simulink model "ultra"  (R2020b)
settings: Solver=FixedStepDiscrete  StartTime=0.0  StopTime=10.0  FixedStep=0.0005  RelTol=1e-3  EnableMultiTasking=on
undefined symbols (not defined in the file): acc_calmax1, acc_calmax2, acc_calmin1, acc_calmin2, akemancanshu, bre, bre_calmax, bre_calmin, ecucoder_acal, I_AN01_5K1, I_AN03_5V, I_AN04_5V, kd, ki, kp, leftmax, O_SW06_HS1A, rightmax, T_add, T_del, tiaoshi, zhiling
libraries: ec5744lib x215, canmsglib x75, simulink x10
(part 7 of 7)

== matlab function ultra/run/ctrl/Subsystem1/control_strategy/MATLAB Function ==
  data: slip_ratio_fl input; torque_cmd_fl output; slip_ratio_fr input; slip_ratio_rl input; slip_ratio_rr input; desired_slip_ratio input; driver_torque_cmd_fl input; driver_torque_cmd_fr input; driver_torque_cmd_rl input; driver_torque_cmd_rr input; dt input; B input; C input; D input; E input; wheel_radius input; torque_cmd_fr output; torque_cmd_rl output; torque_cmd_rr output
function [torque_cmd_fl, torque_cmd_fr, torque_cmd_rl, torque_cmd_rr] = SlipRatioControlWithMagicFormula(slip_ratio_fl, slip_ratio_fr, slip_ratio_rl, slip_ratio_rr, desired_slip_ratio, driver_torque_cmd_fl, driver_torque_cmd_fr, driver_torque_cmd_rl, driver_torque_cmd_rr, dt, B, C, D, E, wheel_radius)

    % 定义持久变量来存储每个轮胎的上一次误差
    persistent e_prev_fl e_prev_fr e_prev_rl e_prev_rr
    if isempty(e_prev_fl)
        e_prev_fl = 0; e_prev_fr = 0; e_prev_rl = 0; e_prev_rr = 0;
    end

    % 滑膜设计参数
    lambda = 2;            
    K = 0.2;               
    delta = 0.05;          

    % 定义一个内部函数来为每个轮胎进行滑膜控制
    function [torque_cmd, e_prev] = singleWheelControl(slip_ratio, desired_slip_ratio, driver_torque_cmd, e_prev, B, C, D, E, wheel_radius)
        % 计算误差和误差的变化率
        e = desired_slip_ratio - slip_ratio;
        e_dot = (e - e_prev) / dt;
        s = e_dot + lambda * e;

        % 使用Magic Formula计算期望的轮胎纵向力
        Fx_desired = D * sin(C * atan(B * desired_slip_ratio - E*(B * desired_slip_ratio - atan(B * desired_slip_ratio))));
        
        % 转换纵向力为期望扭矩
        desired_torque = Fx_desired * wheel_radius;

        % 根据滑模控制策略调整扭矩
        if abs(s) < delta
            torque_adjustment = 0;
        else
            torque_adjustment = K * s;
        end

        % 结合Magic Formula期望扭矩和滑模控制调整来计算输出扭矩
        torque_cmd = desired_torque + torque_adjustment;
        
        % 保证输出扭矩为非负
        torque_cmd = max(0, torque_cmd); 

        % 更新误差以供下次使用
        e_prev = e;
    end

    % 为每个轮胎应用滑模控制策略
    [torque_cmd_fl, e_prev_fl] = singleWheelControl(slip_ratio_fl, desired_slip_ratio, driver_torque_cmd_fl, e_prev_fl, B, C, D, E, wheel_radius);
    [torque_cmd_fr, e_prev_fr] = singleWheelControl(slip_ratio_fr, desired_slip_ratio, driver_torque_cmd_fr, e_prev_fr, B, C, D, E, wheel_radius);
    [torque_cmd_rl, e_prev_rl] = singleWheelControl(slip_ratio_rl, desired_slip_ratio, driver_torque_cmd_rl, e_prev_rl, B, C, D, E, wheel_radius);
    [torque_cmd_rr, e_prev_rr] = singleWheelControl(slip_ratio_rr, desired_slip_ratio, driver_torque_cmd_rr, e_prev_rr, B, C, D, E, wheel_radius);

end

== matlab function ultra/无人TX/转向换算/MATLAB Function1 ==
  data: y1 output; y2 output; biaozhi2 output; baocuo input
function [y1,y2,biaozhi2] = fcn(baocuo)
    persistent i;
     % 初始化状态变量
    if isempty(i)
        i = 1;
    end
    if baocuo==1
        i=1;
    end
    if i<4
        biaozhi2=1;
    else
        biaozhi2=0;
    end
    if mod(i, 2) == 0
        result = 1;
    else
        result = 0;
    end
    
    if result==0
        y1=6307883;
        y2=0;
    else
        y1=6307883;
        y2=128;
    end
    i=i+1;

== matlab function ultra/TX控制器/速度/185右前/MATLAB Function1 ==
  data: v input; T output; a input
function T = fcn(v,a)
% if a>5
%     y = u;
% elseif a>3&&a<5
%     y=1200;
% else
%     y=800;
% end

if v<6000*1.88e-3
    T=2100;
elseif v>11000*1.88e-3
    T=800;
else
    T=1100;
end

== matlab function ultra/RX/287 289右后/Subsystem3/Subsystem/MATLAB Function ==
  data: u input; y output
function y = fcn(u)


y = u/594.06;

== matlab function ultra/TOWORKSTATION/转向/Subsystem/MATLAB Function1 ==
  data: y1 output; y2 output; biaozhi2 output
function [y1,y2,biaozhi2] = fcn()
    persistent i;
     % 初始化状态变量
    if isempty(i)
        i = 1;
    end
    if i<16
        biaozhi2=1;
    else
        biaozhi2=0;
    end
    if mod(i, 2) == 0
        result = 1;
    else
        result = 0;
    end
    
    if result==0
        y1=6307883;
        y2=0;
    else
        y1=6307883;
        y2=128;
    end
    i=i+1;

== matlab function ultra/TX控制器/速度/184左前/MATLAB Function ==
  data: u input; y output; zhidongesc input; zhidongebs input
function y = fcn(u,zhidongesc,zhidongebs)
 y = u*594.06;
if zhidongesc>1800&&zhidongebs==2
    y = u*594.06;
end
if zhidongesc<1500&&zhidongebs==2
    y=0;
end

== matlab function ultra/TX控制器/速度/185右前/MATLAB Function ==
  data: u input; y output; zhidongesc input; zhidongebs input
function y = fcn(u,zhidongesc,zhidongebs)
 y = u*594.06;
if zhidongesc>1800&&zhidongebs==2
    y = u*594.06;
end
if zhidongesc<1500&&zhidongebs==2
    y=0;
end

== matlab function ultra/TX控制器/速度/189左后/MATLAB Function ==
  data: u input; y output; zhidongesc input; zhidongebs input
function y = fcn(u,zhidongesc,zhidongebs)
 y = u*594.06;
if zhidongesc>1800&&zhidongebs==2
    y = u*594.06;
end
if zhidongesc<1500&&zhidongebs==2
    y=0;
end

== matlab function ultra/TX控制器/速度/185右前/MATLAB Function3 ==
  data: v input; y output; angle input; vz input; model input
function y = fcn(v, angle, vz,model)
if (angle>3||angle<-3)&&model==3%4650000,4870000,4741002
    y=vz*594.06;
else
    y = v;
end

== matlab function ultra/run/滑移率计算 ==
  data: vyouhou input; slipyuohou output; vyouqian input; vzouhou input; vzuoqian input; v input; slipyouqian output; slipzuohou output; slipzuoqian output; vmin input
function [slipyuohou,slipyouqian,slipzuohou,slipzuoqian] = fcn(vyouhou,vyouqian,vzouhou,vzuoqian,v,vmin)

    v1=vmin;
if v<0.1
    v1 = vmin;
else
    v1 = v;
end
slipyuohou= (vyouhou - v1) / vyouhou;
slipzuohou= (vzouhou - v1) / vzouhou;
slipyouqian= (vyouqian - v1) / vyouqian;
slipzuoqian= (vzuoqian - v1) / vzuoqian;
end

== matlab function ultra/TOWORKSTATION/转向/Subsystem/Subsystem/MATLAB Function ==
  data: steer output; y output
function [steer,y] = fcn()
  persistent i;
     % 初始化状态变量
    if isempty(i)
        i = 0;
    end
    x=0;
    if i>1
       steer=62000* sin(2 * pi * i)+683198;
%            steer= 3494 *x+2.407e+04 ;
%            x=(i-1)*50;
%            if i>8.2
%                i=1;
%            end
    else
        steer=683198
    end
%     if i>0.2     
%         steer=  3271 *x+6.821e+05 ;
% %         if x==0
% %             steer=25092;
% %         end
%     else
%         steer=683198;
%     end
    i=i+0.02;
  persistent time;
     % 初始化状态变量
    if isempty(time)
        time = 0;
    end
    if mod(time, 2) == 0
        result = 1;
    else
        result = 0;
    end
    if time<5
    y=6;
 
    elseif time>=5&&time<10
    y=15;
  
    elseif time>=10
        if result==1
            y=79;
        else
            y=63;
        end
    else
        y=6;
    end   
    time=time+1;
    if time>650
        y=6;
    end
end

== matlab function ultra/TX控制器/MATLAB Function1 ==
  data: y output; model input
function y = fcn(model)
if (model==1||model==2||model==3||model==4||model==5||model==6||model==7||model==8)
    y=1;
else
    y=0;
end

== matlab function ultra/run/ctrl/Subsystem1/control_strategy/差速/差速/pid ==
  data: v input; u input; v_zuoqian output
function v_zuoqian  = carPIDControl(v, u)
    % 赛车PID控制器参数
    kp = 0.2;
    ki = 0.1;
    kd = 0.01;
    
    % 状态变量
    persistent integral previous_error 
    
    % 初始化状态变量
    if isempty(integral)
        integral = 0;
        previous_error = 0;
        i=0;
    end
    
    % PID控制器计算
    error = u - v;
    integral = integral + error*0.02;
    derivative = (error - previous_error)/0.02;
    
        if integral > 0.4    
        integral = 0.4;
        end
        if integral < -0.4    
        integral = -0.4;
        end
    
   v_zuoqian = kp * error + ki * integral + kd * derivative;
   
    % 保存上一个误差用于下次计算
    previous_error = error;
end

== matlab function ultra/run/ctrl/Subsystem1/control_strategy/差速/差速/pid1 ==
  data: v input; u input; v_zuoqian output
function v_zuoqian  = carPIDControl(v, u)
    % 赛车PID控制器参数
    kp = 0.2;
    ki = 0.1;
    kd = 0.01;
    
    % 状态变量
    persistent integral previous_error 
    
    % 初始化状态变量
    if isempty(integral)
        integral = 0;
        previous_error = 0;
        i=0;
    end
    
    % PID控制器计算
    error = u - v;
    integral = integral + error*0.02;
    derivative = (error - previous_error)/0.02;
    
        if integral > 0.4    
        integral = 0.4;
        end
        if integral < -0.4    
        integral = -0.4;
        end
    
   v_zuoqian = kp * error + ki * integral + kd * derivative;
   
    % 保存上一个误差用于下次计算
    previous_error = error;
end

== matlab function ultra/run/ctrl/Subsystem1/control_strategy/差速/差速/pid2 ==
  data: v input; u input; v_zuoqian output
function v_zuoqian  = carPIDControl(v, u)
    % 赛车PID控制器参数
    kp = 0.2;
    ki = 0.1;
    kd = 0.01;
    
    % 状态变量
    persistent integral previous_error 
    
    % 初始化状态变量
    if isempty(integral)
        integral = 0;
        previous_error = 0;
        i=0;
    end
    
    % PID控制器计算
    error = u - v;
    integral = integral + error*0.02;
    derivative = (error - previous_error)/0.02;
    
        if integral > 0.4    
        integral = 0.4;
        end
        if integral < -0.4    
        integral = -0.4;
        end
    
   v_zuoqian = kp * error + ki * integral + kd * derivative;
   
    % 保存上一个误差用于下次计算
    previous_error = error;
end

== matlab function ultra/run/ctrl/Subsystem1/control_strategy/差速/差速/pid3 ==
  data: v input; u input; v_zuoqian output
function v_zuoqian  = carPIDControl(v, u)
    % 赛车PID控制器参数
    kp = 0.2;
    ki = 0.1;
    kd = 0.01;
    
    % 状态变量
    persistent integral previous_error 
    
    % 初始化状态变量
    if isempty(integral)
        integral = 0;
        previous_error = 0;
        i=0;
    end
    
    % PID控制器计算
    error = u - v;
    integral = integral + error*0.02;
    derivative = (error - previous_error)/0.02;
    
        if integral > 0.4    
        integral = 0.4;
        end
        if integral < -0.4    
        integral = -0.4;
        end
    
   v_zuoqian = kp * error + ki * integral + kd * derivative;
   
    % 保存上一个误差用于下次计算
    previous_error = error;
end

== matlab function ultra/TX控制器/速度/184左前/MATLAB Function3 ==
  data: v input; y output; angle input; vz input; model input
function y = fcn(v, angle, vz,model)
if(angle>3||angle<-3)&&model==3%4650000,4870000,4741002
    y=vz*594.06;
else
    y = v;
end

== matlab function ultra/run/ctrl/Subsystem1/control_strategy/差速/差速/阿克曼转向 ==
  data: wfl output; v input; wfr output; wrl output; wrr output; a input; angle input
function [wfl,wfr,wrl,wrr]= fcn(v,a,angle)
%22e轴距：1170mm 轮距 1530mm 前47%后53%即，前0.72后0.81 
L=1.53;%前后轴距    u是转角
d=1.17;%车宽
c1=0.93;%前车对角线的一半
c2=1;
k=1;%12.641传动比

Rcg=v^2/a;
if angle<0
    Rfr=sqrt(c1^2+Rcg^2-2*c1*Rcg*cos(2.25));
    Rfl=sqrt(c1^2+Rcg^2-2*c1*Rcg*cos(0.89));
    Rrl=sqrt(c2^2+Rcg^2-2*c2*Rcg*cos(0.945));
    Rrr=sqrt(c2^2+Rcg^2-2*c2*Rcg*cos(2.2));
    wfl=k*v/Rcg*Rfl;
    wfr=k*v/Rcg*Rfr;
    wrl=k*v/Rcg*Rrl;
    wrr=k*v/Rcg*Rrr;
else
    Rfl=sqrt(c1^2+Rcg^2-2*c1*Rcg*cos(2.25));
    Rfr=sqrt(c1^2+Rcg^2-2*c1*Rcg*cos(0.89));
    Rrr=sqrt(c2^2+Rcg^2-2*c2*Rcg*cos(0.945));
    Rrl=sqrt(c2^2+Rcg^2-2*c2*Rcg*cos(2.2));
    wfl=k*v/Rcg*Rfl;
    wfr=k*v/Rcg*Rfr;
    wrl=k*v/Rcg*Rrl;
    wrr=k*v/Rcg*Rrr; 
end
wfl=594.06*min(wfl,v+2);
wfr=594.06*min(wfr,v+2);
wrl=594.06*min(wrl,v+2);
wrr=594.06*min(wrr,v+2);
wfl=594.06*max(wfl,v-2);
wfr=594.06*max(wfr,v-2);
wrl=594.06*max(wrl,v-2);
wrr=594.06*max(wrr,v-2);

== matlab function ultra/TX控制器/速度/188右后/MATLAB Function ==
  data: u input; y output; zhidongesc input; zhidongebs input
function y = fcn(u,zhidongesc,zhidongebs)
 y = u*594.06;
if zhidongesc>1800&&zhidongebs==2
    y = u*594.06;
end
if zhidongesc<1500&&zhidongebs==2
    y=0;
end
